simulink model "passiveCellBalancing"  (R2023a)
settings: Solver=VariableStepAuto  StartTime=0.0  StopTime=3500  RelTol=1e-3
undefined symbols (not defined in the file): Ion, Lithium
libraries: spsBatteryLib x3, spsMosfetLib x3, spsSeriesRLCBranchLib x3, sps_lib x1
settings Model: Creator=DELL  LastModifiedBy=DELL

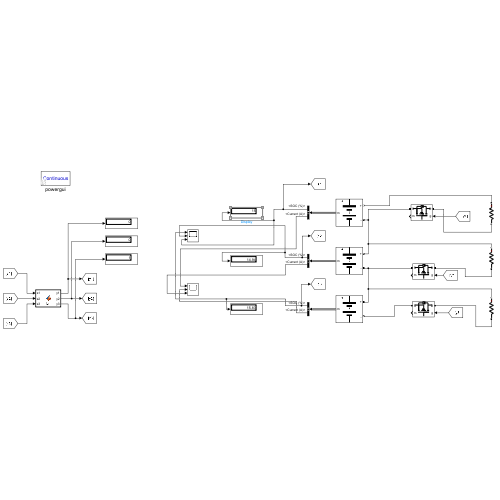
[thumbnail: Simulink's stored preview of the top-level diagram]
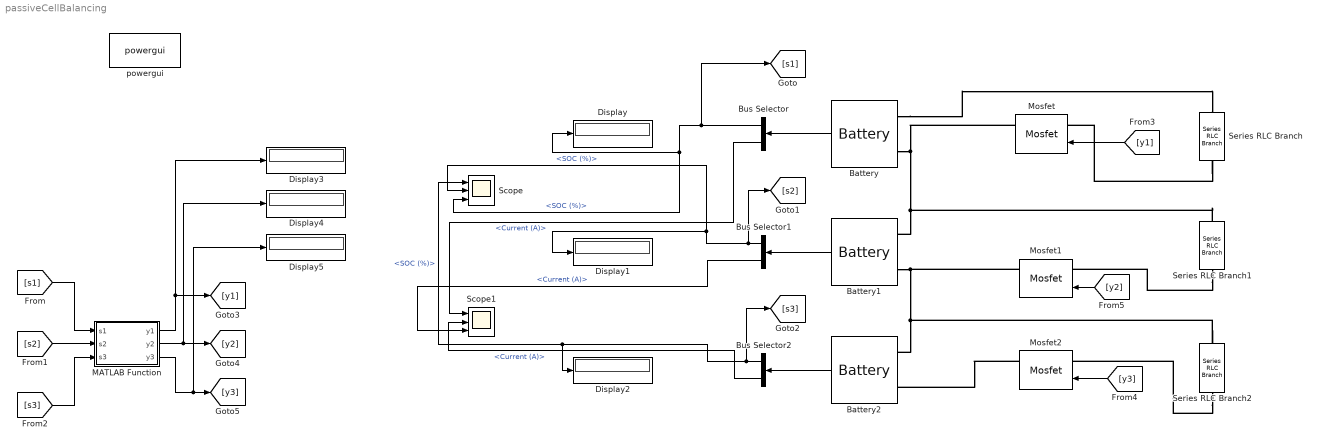
== system passiveCellBalancing ==
  Battery : spsBatteryLib/Battery  BatType=Lithium-Ion  ShowTempParam=off  ThermalPreset=no  ShowAgeParam=off  NomV=7.2  NomQ=5.4  SOC=15  Batt_Tr=30  PresetModel=on  MaxQ=5.4  MinV=5.4  FullV=8.3807  Dis_rate=2.3478  R=0.013333  Normal_OP=4.8835  expZone="[7.7788      0.2653]"  current=[6.5 13 32.5]  Units=Time  Tci=20  NomT=20  T2=-30  MaxQ2=4.8  FullV2=7.1  Normal_OP2=5.655  expZone2="[6.58           1]"  Rca=0.6  ti=2000  Dp=0  Neq0=0  Tsim=1e6  Ta1=25  Qeol=5.4*0.9  Reol=0.013333*1.2  Char_age=[2.3478, 3]  Dis_age=[2.3478, 10]  N1=1500  N2=10500  N3=1000  N4=1400  Ta2=45  N5=950
  Battery1 : spsBatteryLib/Battery  BatType=Lithium-Ion  ShowTempParam=off  ThermalPreset=no  ShowAgeParam=off  NomV=7.2  NomQ=5.4  SOC=30  Batt_Tr=30  PresetModel=on  MaxQ=5.4  MinV=5.4  FullV=8.3807  Dis_rate=2.3478  R=0.013333  Normal_OP=4.8835  expZone="[7.7788      0.2653]"  current=[6.5 13 32.5]  Units=Time  Tci=20  NomT=20  T2=-30  MaxQ2=4.8  FullV2=7.1  Normal_OP2=5.655  expZone2="[6.58           1]"  Rca=0.6  ti=2000  Dp=0  Neq0=0  Tsim=1e6  Ta1=25  Qeol=5.4*0.9  Reol=0.013333*1.2  Char_age=[2.3478, 3]  Dis_age=[2.3478, 10]  N1=1500  N2=10500  N3=1000  N4=1400  Ta2=45  N5=950
  Battery2 : spsBatteryLib/Battery  BatType=Lithium-Ion  ShowTempParam=off  ThermalPreset=no  ShowAgeParam=off  NomV=7.2  NomQ=5.4  SOC=60  Batt_Tr=30  PresetModel=on  MaxQ=5.4  MinV=5.4  FullV=8.3807  Dis_rate=2.3478  R=0.013333  Normal_OP=4.8835  expZone="[7.7788      0.2653]"  current=[6.5 13 32.5]  Units=Time  Tci=20  NomT=20  T2=-30  MaxQ2=4.8  FullV2=7.1  Normal_OP2=5.655  expZone2="[6.58           1]"  Rca=0.6  ti=2000  Dp=0  Neq0=0  Tsim=1e6  Ta1=25  Qeol=5.4*0.9  Reol=0.013333*1.2  Char_age=[2.3478, 3]  Dis_age=[2.3478, 10]  N1=1500  N2=10500  N3=1000  N4=1400  Ta2=45  N5=950
  Bus Selector : BusSelector  OutputSignals=SOC (%),Current (A)
  Bus Selector1 : BusSelector  OutputSignals=SOC (%),Current (A)
  Bus Selector2 : BusSelector  OutputSignals=SOC (%),Current (A)
  Display{,1..5} (6 alike) : Display
  MATLAB Function : MATLAB Function  TreatAsAtomicUnit=on
  Mosfet : spsMosfetLib/Mosfet  Ron=0.1  Lon=0  Rd=0.01  Vfd=0  IC=0  Rs=1e5  Cs=inf  Measurements=on
  Mosfet1 : spsMosfetLib/Mosfet  Ron=0.1  Lon=0  Rd=0.01  Vfd=0  IC=0  Rs=1e5  Cs=inf  Measurements=on
  Mosfet2 : spsMosfetLib/Mosfet  Ron=0.1  Lon=0  Rd=0.01  Vfd=0  IC=0  Rs=1e5  Cs=inf  Measurements=on
  Scope : Scope  NumInputPorts=3
  Scope1 : Scope  NumInputPorts=3
  Series RLC Branch : spsSeriesRLCBranchLib/Series RLC Branch  LConnTagsString=__new0  RConnTagsString=__new0  BranchType=R  Resistance=3  Inductance=1e-3  SetiL0=off  InitialCurrent=0  Capacitance=1e-6  Setx0=off  InitialVoltage=0  Measurements=None
  Series RLC Branch1 : spsSeriesRLCBranchLib/Series RLC Branch  LConnTagsString=__new0  RConnTagsString=__new0  BranchType=R  Resistance=3  Inductance=1e-3  SetiL0=off  InitialCurrent=0  Capacitance=1e-6  Setx0=off  InitialVoltage=0  Measurements=None
  Series RLC Branch2 : spsSeriesRLCBranchLib/Series RLC Branch  LConnTagsString=__new0  RConnTagsString=__new0  BranchType=R  Resistance=3  Inductance=1e-3  SetiL0=off  InitialCurrent=0  Capacitance=1e-6  Setx0=off  InitialVoltage=0  Measurements=None
  powergui : sps_lib/powergui  Priority=1  SimulationMode=Continuous  SampleTime=50e-6  frequency=60  Iterations=50  frequencyindice=0  Pbase=100e6  ErrMax=1e-4  UnitsV=kV  UnitsW=MW  buscounter=0  FunctionMessages=off  echomessages=off  EnableUseOfTLC=off  CurrentSourceSwitches=off  DisableSnubberDevices=off  DisableRonSwitches=off  DisableVfSwitches=off  DisplayEquations=off  AutomaticDiscreteSolvers=off  SolverType=Tustin/Backward Euler (TBE)  Interpol=off  ExternalGateDelay=off  methode=off  Ts=100  x0status=blocks  SPID=on  SwTol=0  HookPort=off  NonlinearTolerance=1e-4  nMaxIteration=100  ContinueOnMaxIteration=off  RestoreLinks=warning  ResistiveCurrentMeasurement=off  Frange=[0:2:500]  Ylog=off  Xlog=on  ShowGrid=off  save=off  variable=ZData  structure=0  ZoomFFT=off  StartTime=0.0  cycles=1  DisplayStyle=1  fundamental=60  FreqAxis=off  MaxFrequency=1000  frequencyindicesteady=1  RmsSteady=1  display=off
  wires:
  Battery/1 -> Bus Selector/1
  Battery1/1 -> Bus Selector1/1
  Battery2/1 -> Bus Selector2/1
  Bus Selector/1 -> [s1], Display/1, Scope/3  "<SOC (%)>"
  Bus Selector1/1 -> [s2], Display1/1, Scope/2  "<SOC (%)>"
  Bus Selector2/1 -> [s3], Display2/1, Scope/1  "<SOC (%)>"
  Bus Selector/2 -> Scope1/1  "<Current (A)>"
  Bus Selector1/2 -> Scope1/3  "<Current (A)>"
  Bus Selector2/2 -> Scope1/2  "<Current (A)>"
  [s2] -> MATLAB Function/2(s2)
  [s1] -> MATLAB Function/1(s1)
  [s3] -> MATLAB Function/3(s3)
  MATLAB Function/1(y1) -> Display3/1, [y1]
  MATLAB Function/2(y2) -> Display4/1, [y2]
  MATLAB Function/3(y3) -> Display5/1, [y3]
  [y2] -> Mosfet1/1
  [y3] -> Mosfet2/1
  [y1] -> Mosfet/1
  connections:
  Battery/LConn2 -- Mosfet/RConn1 -- Series RLC Branch1/LConn1 -- Battery1/LConn1
  Battery1/LConn2 -- Mosfet1/RConn1 -- Series RLC Branch2/LConn1 -- Battery2/LConn1
  Battery/LConn1 -- Series RLC Branch/LConn1
  Series RLC Branch/RConn1 -- Mosfet/LConn1
  Series RLC Branch1/RConn1 -- Mosfet1/LConn1
  Series RLC Branch2/RConn1 -- Mosfet2/LConn1
  Mosfet2/RConn1 -- Battery2/LConn2

== matlab function passiveCellBalancing/MATLAB Function ==
  data: s1 input; y1 output; s2 input; s3 input; y2 output; y3 output
function [y1, y2, y3]= fcn(s1, s2, s3)
s1 = int16(s1);
s2 = int16(s2);
s3 = int16(s3);

a = min([s1 s2 s3]);
if(s1 == a)
    if (s1 == a && s2 == a)
        y1 = 0;
        y2 = 0;
        y3 = 1;
    elseif (s1 == a && s3 == a)
        y1 = 0;
        y2 = 1;
        y3 = 0;
    elseif (s1 == a)
        y1 = 0;
        y2 = 1;
        y3 = 1;
    else 
        y1 = 0;
        y2 = 0;
        y3 = 0;
    end
elseif(s2==a)
    if(s2==a && s3==a)
        y1 = 1;
        y2 = 0;
        y3 = 0;
    elseif (s2 == a && s1 == a)
        y1 = 0;
        y2 = 0;
        y3 = 1;
    elseif (s2 == a)
        y1 = 1;
        y2 = 0;
        y3 = 1;
    else 
        y1 = 0;
        y2 = 0;
        y3 = 0;
    end
elseif(s3==a)
    if(s3==a && s2==a)
        y1 = 1;
        y2 = 0;
        y3 = 0;
    elseif (s3 == a && s1 == a)
        y1 = 0;
        y2 = 1;
        y3 = 0;
    elseif (s3 == a)
        y1 = 1;
        y2 = 1;
        y3 = 0;
    else 
        y1 = 0;
        y2 = 0;
        y3 = 0;
    end
else
    y1 = 0;
    y2 = 0;
    y3 = 0;
end
